simulink model "Load_control_NLMPC"  (R2021a)
settings: Solver=FixedStepAuto  StartTime=0.0  StopTime=10  FixedStep=0.08  RelTol=1e-3  EnableMultiTasking=on
libraries: mpclib x1, simulink x1
(part 1 of 2)
settings Model: ExtModeAutoUpdateStatusClock=off  Creator=benoit  LastModifiedBy=norouziy
settings SolverCC: AlgebraicLoopSolver=TrustRegion
settings DataIOCC: LimitDataPoints=on  SaveFormat=Array  SignalLoggingSaveFormat=ModelDataLogs  SignalLoggingName=sigsOut
settings OptimizationCC: InitFltsAndDblsToZero=on  LifeSpan=inf
settings DebuggingCC: SaveWithParameterizedLinksMsg=none  UnderspecifiedInitializationDetection=Classic  MergeDetectMultiDrivingBlocksExec=none  SignalResolutionControl=TryResolveAllWithWarning  MultiTaskDSMMsg=warning  MultiTaskCondExecSysMsg=none  FcnCallInpInsideContextMsg=warning  SFUnexpectedBacktrackingDiag=warning  SFNoUnconditionalDefaultTransitionDiag=warning  SFExecutionAtInitializationDiag=none  SFMachineParentedDataDiag=warning  ArithmeticOperatorsInVariantConditions=warning
settings HardwareCC: ProdBitPerPointer=32  ProdBitPerSizeT=32  ProdBitPerPtrDiffT=32  ProdLargestAtomicFloat=None  ProdIntDivRoundTo=Undefined  ProdEndianess=Unspecified  ProdWordSize=32  ProdHWDeviceType=32-bit Generic  TargetHWDeviceType=32-bit Generic  TargetUnknown=on  ProdEqTarget=off
settings ModelReferenceCC: PropagateSignalLabelsOutOfModel=off
settings SFSimCC: SimUseLocalCustomCode=off  CustomCodeUndefinedFunction=UseInterfaceOnly
settings RTWCC: RTWUseLocalCustomCode=off
settings CodeAppCC: StateflowObjectComments=on
settings GRTTargetCC: TargetFcnLib=ansi_tfl_tmw.mat  TargetLangStandard=C89/C90 (ANSI)  CombineOutputUpdateFcns=off  GRTInterface=on
settings ConfigComp: CovMetricSettings=dw  CovSaveCumulativeToWorkspaceVar=on  CovSaveSingleToWorkspaceVar=on

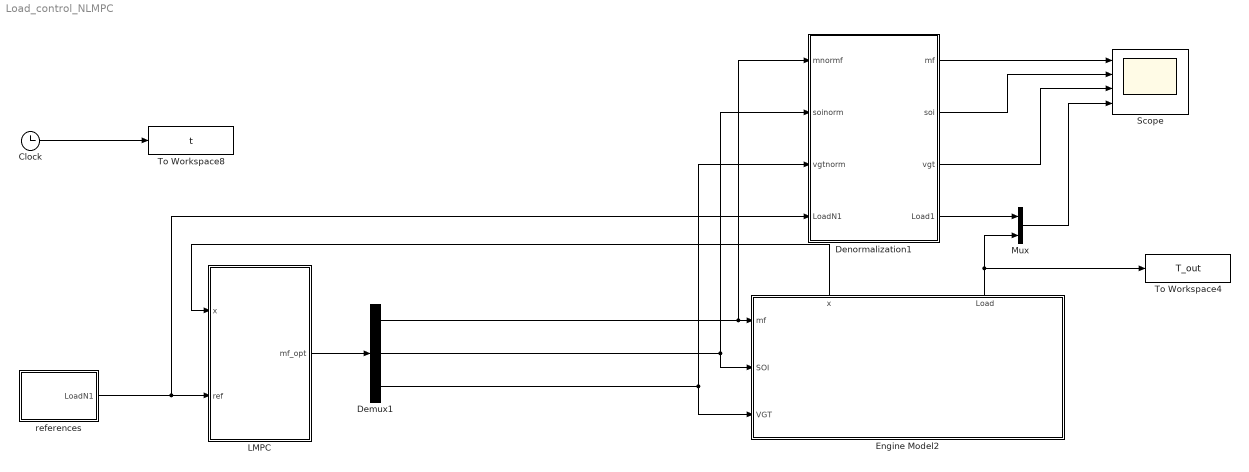
== system Load_control_NLMPC ==
  Clock : Clock
  Demux1 : Demux  Outputs=3
  Denormalization1 : Subsystem
  Engine Model2 : Subsystem
      settings: PortSchema="{\"entries\":[{\"content\":{\"sides\":[{\"content\":{\"connectorIds\":[\"In1\",\"In2\",\"In3\"]},\"type\":\"ConnectorPlacement.EquallySpacedRectSide\",\"uuid\":\"aed6c330-d322-4273-ac99-0d57e7c0b354\"},{\"content\":{\"connectorIds\":[],\"side\":\"RIGHT\"},\"type\":\"ConnectorPlacement.EquallySpacedRectSide\",\"uuid\":\"4fbb33cf-927e-40a8-96e5-fef56b1fca2a\"},{\"content\":{\"connectorIds\":[\"Out1\",\"Out2\"],\"side\":\"TOP\"},\"type\":\"ConnectorPlacement.EquallySpacedRectSide\",\"uuid\":\"48b318f3-0e1e-4e5f-9557-fff2a225800a\"}]},\"type\":\"ConnectorPlacement.EquallySpacedConnector\",\"uuid\":\"6084b50f-4a7b-42af-a0f6-342c5d597c67\"}],\"packageUris\":[\"http://schema.mathworks.com/mf0/Connector/R2020b\"],\"version\":\"1.0\"}"
  LMPC : Subsystem
  Mux : Mux  Inputs=2
  Scope : Scope  NumInputPorts=4
  To Workspace4 : ToWorkspace  VariableName=T_out  SaveFormat=Timeseries  SampleTime=-1
  To Workspace8 : ToWorkspace  VariableName=t  SaveFormat=Timeseries  SampleTime=-1
  references : Subsystem
  wires:
  Clock/1 -> To Workspace8/1
  Demux1/1 -> Denormalization1/1(mnormf), Engine Model2/1(mf)
  references/1(LoadN1) -> Denormalization1/4(LoadN1), LMPC/2(ref)
  LMPC/1(mf_opt) -> Demux1/1
  Demux1/3 -> Denormalization1/3(vgtnorm), Engine Model2/3(VGT)
  Demux1/2 -> Denormalization1/2(soinorm), Engine Model2/2(SOI)
  Mux/1 -> Scope/4
  Engine Model2/2(Load) -> To Workspace4/1, Mux/2
  Engine Model2/1(x) -> LMPC/1(x)
  Denormalization1/1(mf) -> Scope/1
  Denormalization1/2(soi) -> Scope/2
  Denormalization1/3(vgt) -> Scope/3
  Denormalization1/4(Load1) -> Mux/1

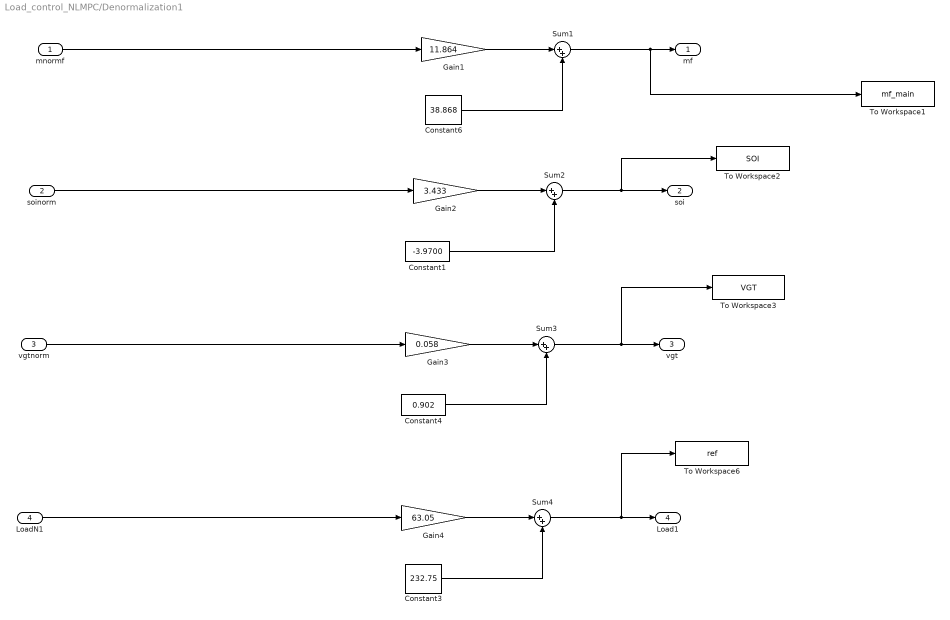
== system Load_control_NLMPC/Denormalization1 ==
  mnormf : Inport
  soinorm : Inport  Port=2
  vgtnorm : Inport  Port=3
  LoadN1 : Inport  Port=4
  Constant1 : Constant  Value=-3.9700
  Constant3 : Constant  Value=232.75
  Constant4 : Constant  Value=0.902
  Constant6 : Constant  Value=38.868
  Gain1 : Gain  Gain=11.864
  Gain2 : Gain  Gain=3.433
  Gain3 : Gain  Gain=0.058
  Gain4 : Gain  Gain=63.05
  Sum{1..4} (4 alike) : Sum  Inputs=|++
  To Workspace1 : ToWorkspace  VariableName=mf_main  SaveFormat=Timeseries  SampleTime=-1
  To Workspace2 : ToWorkspace  VariableName=SOI  SaveFormat=Timeseries  SampleTime=-1
  To Workspace3 : ToWorkspace  VariableName=VGT  SaveFormat=Timeseries  SampleTime=-1
  To Workspace6 : ToWorkspace  VariableName=ref  SaveFormat=Timeseries  SampleTime=-1
  mf : Outport
  soi : Outport  Port=2
  vgt : Outport  Port=3
  Load1 : Outport  Port=4
  wires:
  mnormf/1 -> Gain1/1
  Gain1/1 -> Sum1/1
  Constant6/1 -> Sum1/2
  Constant1/1 -> Sum2/2
  soinorm/1 -> Gain2/1
  Gain2/1 -> Sum2/1
  Sum3/1 -> To Workspace3/1, vgt/1
  Constant4/1 -> Sum3/2
  vgtnorm/1 -> Gain3/1
  Gain3/1 -> Sum3/1
  LoadN1/1 -> Gain4/1
  Gain4/1 -> Sum4/1
  Sum4/1 -> To Workspace6/1, Load1/1
  Constant3/1 -> Sum4/2
  Sum2/1 -> To Workspace2/1, soi/1
  Sum1/1 -> To Workspace1/1, mf/1

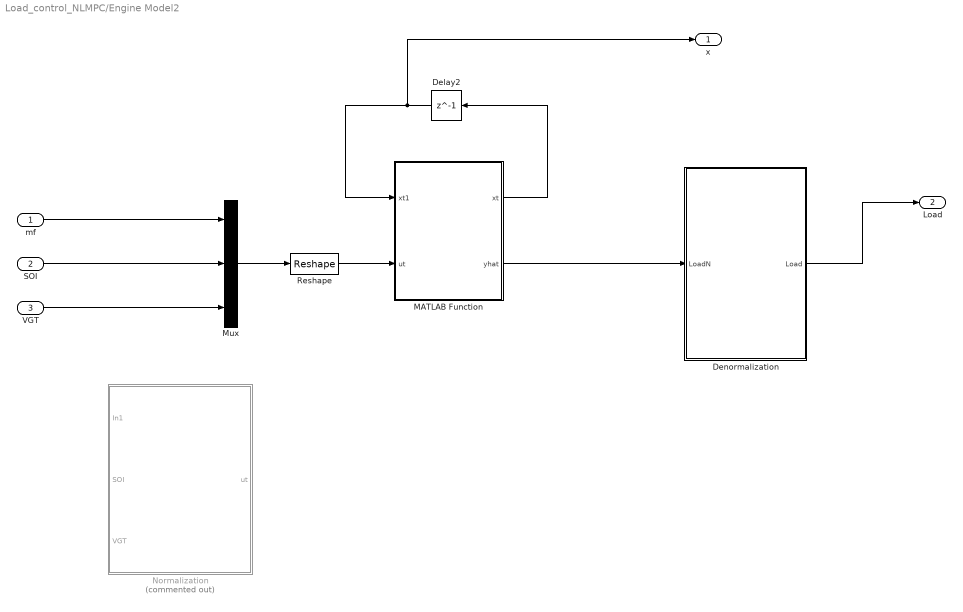
== system Load_control_NLMPC/Engine Model2 ==
  mf : Inport
  SOI : Inport  Port=2
  VGT : Inport  Port=3
  Delay2 : Delay  DelayLength=1  InitialCondition=zeros(53,1)
  Denormalization : Subsystem
  MATLAB Function : MATLAB Function  TreatAsAtomicUnit=on
  Mux : Mux  Inputs=3
  Normalization : Subsystem  Commented=on
  Reshape : Reshape  OutputDimensionality=Customize  OutputDimensions=[3,1]
  x : Outport
  Load : Outport  Port=2
  wires:
  MATLAB Function/1(xt) -> Delay2/1
  Delay2/1 -> x/1, MATLAB Function/1(xt1)
  Denormalization/1(Load) -> Load/1
  Mux/1 -> Reshape/1
  mf/1 -> Mux/1
  SOI/1 -> Mux/2
  VGT/1 -> Mux/3
  MATLAB Function/2(yhat) -> Denormalization/1(LoadN)
  Reshape/1 -> MATLAB Function/2(ut)

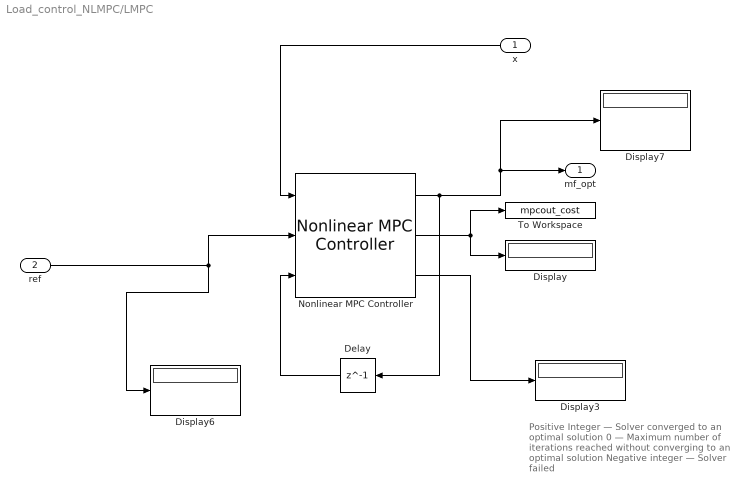
== system Load_control_NLMPC/LMPC ==
  note: Positive Integer — Solver converged to an optimal solution
      | 0 — Maximum number of iterations reached without converging to an optimal solution
      | Negative integer — Solver failed
  x : Inport
  ref : Inport  Port=2
  Delay : Delay  DelayLength=1
  Display{,3,6..7} (4 alike) : Display
  Nonlinear MPC Controller : mpclib/Nonlinear MPC Controller  SCDEnableBlockLinearizationSpecification=on  nlmpcobj=nlobj  UseObjectTs=on  UseMEX=off  md_enabled=off  mvtarget_enabled=off  param_enabled=off  cost_enabled=on  mvseq_enabled=off  stateseq_enabled=off  ovseq_enabled=off  slack_enabled=off  status_enabled=on  ov_min=off  ov_max=off  mv_min=off  mv_max=off  mvrate_min=off  mvrate_max=off  state_min=off  state_max=off  ov_weight=off  mv_weight=off  mvrate_weight=off  ecr_weight=off  nlp_initialize=off
  To Workspace : ToWorkspace  VariableName=mpcout_cost  SaveFormat=Timeseries  SampleTime=-1
  mf_opt : Outport
  wires:
  Nonlinear MPC Controller/1 -> Delay/1, Display7/1, mf_opt/1
  x/1 -> Nonlinear MPC Controller/1
  ref/1 -> Nonlinear MPC Controller/2, Display6/1
  Nonlinear MPC Controller/2 -> Display/1, To Workspace/1
  Nonlinear MPC Controller/3 -> Display3/1
  Delay/1 -> Nonlinear MPC Controller/3

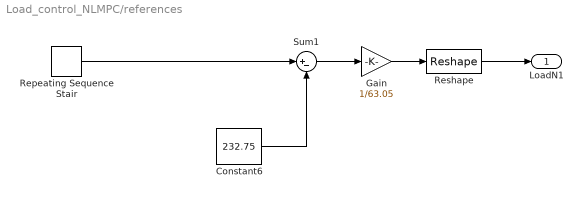
== system Load_control_NLMPC/references ==
  Constant6 : Constant  Value=232.75
  Gain : Gain  Gain=1/63.05
  Repeating Sequence Stair : simulink/Sources/Repeating Sequence Stair  OutValues=load_ref  tsamp=-1  OutMin=[]  OutMax=[]  OutDataTypeStr=double  OutputDataTypeScalingMode=double  OutDataType=fixdt(0,8)  ConRadixGroup=Best Precision: Vector-wise  OutScaling=2^-12
  Reshape : Reshape  OutputDimensionality=Customize
  Sum1 : Sum  Inputs=|+-
  LoadN1 : Outport
  wires:
  Reshape/1 -> LoadN1/1
  Constant6/1 -> Sum1/2
  Sum1/1 -> Gain/1
  Repeating Sequence Stair/1 -> Sum1/1
  Gain/1 -> Reshape/1

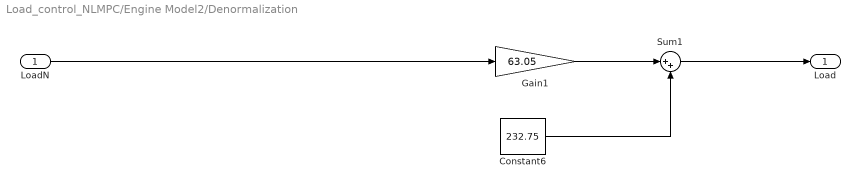
== system Load_control_NLMPC/Engine Model2/Denormalization ==
  LoadN : Inport
  Constant6 : Constant  Value=232.75
  Gain1 : Gain  Gain=63.05
  Sum1 : Sum  Inputs=|++
  Load : Outport
  wires:
  LoadN/1 -> Gain1/1
  Sum1/1 -> Load/1
  Gain1/1 -> Sum1/1
  Constant6/1 -> Sum1/2

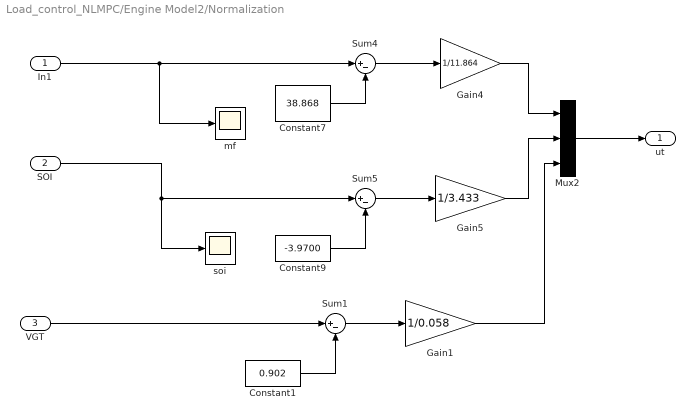
== system Load_control_NLMPC/Engine Model2/Normalization ==
  In1 : Inport
  SOI : Inport  Port=2
  VGT : Inport  Port=3
  Constant1 : Constant  Value=0.902
  Constant7 : Constant  Value=38.868
  Constant9 : Constant  Value=-3.9700
  Gain1 : Gain  Gain=1/0.058
  Gain4 : Gain  Gain=1/11.864
  Gain5 : Gain  Gain=1/3.433
  Mux2 : Mux  Inputs=3
  Sum1 : Sum  Inputs=|+-
  Sum4 : Sum  Inputs=|+-
  Sum5 : Sum  Inputs=|+-
  mf : Scope
  soi : Scope
  ut : Outport
  wires:
  Gain4/1 -> Mux2/1
  SOI/1 -> soi/1, Sum5/1
  In1/1 -> mf/1, Sum4/1
  Sum4/1 -> Gain4/1
  Gain5/1 -> Mux2/2
  Constant9/1 -> Sum5/2
  Sum5/1 -> Gain5/1
  Constant7/1 -> Sum4/2
  Mux2/1 -> ut/1
  Sum1/1 -> Gain1/1
  Constant1/1 -> Sum1/2
  VGT/1 -> Sum1/1
  Gain1/1 -> Mux2/3
